simulink model "encoder_Test_typeII"  (R2021b)
settings: Solver=FixedStepAuto  StartTime=0.0  StopTime=300  FixedStep=0.005  RelTol=1e-3  EnableMultiTasking=on
libraries: raspberrypiCommlib x5
settings Model: Creator=The MathWorks, Inc.  LastModifiedBy=kboxi
settings SolverCC: AlgebraicLoopSolver=TrustRegion  PositivePriorityOrder=on
settings OptimizationCC: EnhancedBackFolding=on  PassReuseOutputArgsThreshold=0  MaxStackSize=64  OptimizeBlockOrder=speed  DifferentSizesBufferReuse=on  OptimizationCustomize=off
settings DebuggingCC: ParameterTunabilityLossMsg=error  SFMachineParentedDataDiag=warning
settings HardwareCC: ProdBitPerPointer=32  ProdBitPerSizeT=32  ProdBitPerPtrDiffT=32  ProdLargestAtomicInteger=Long  ProdLargestAtomicFloat=Double  ProdWordSize=32  ProdLongLongMode=on  ProdHWDeviceType=ARM Compatible->ARM Cortex  UseEmbeddedCoderFeatures=off
settings RTWCC: Description=Embedded Coder  SystemTargetFile=ert.tlc  HardwareBoard=Raspberry Pi  TLCOptions="-aInlineSetEventsForThisBaseRateFcn=TLC_FALSE -aSuppressMultiTaskScheduler=TLC_FALSE  -aRateBasedStepFcn=0"  TemplateMakefile=ert_default_tmf  Toolchain=GNU GCC Embedded Linux  BuildConfiguration=Faster Runs
settings CodeAppCC: ForceParamTrailComments=on  OperatorAnnotations=on
settings ERTTargetCC: ERTCustomFileBanners=off  SupportContinuousTime=on  SupportNonInlinedSFcns=on  RemoveResetFunc=off  SupportVariableSizeSignals=on  ModelStepFunctionPrototypeControlCompliant=off  ExtModeTransport=2  ExtModeStaticAlloc=on  ExtModeMexFile=ext_xcp  ExtModeIntrfLevel=Level2 - Open

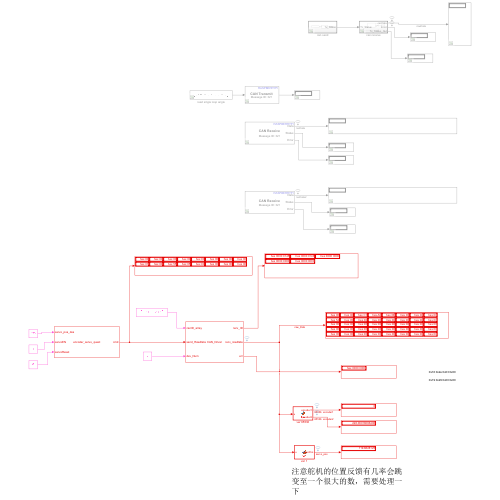
[thumbnail: Simulink's stored preview of the top-level diagram]
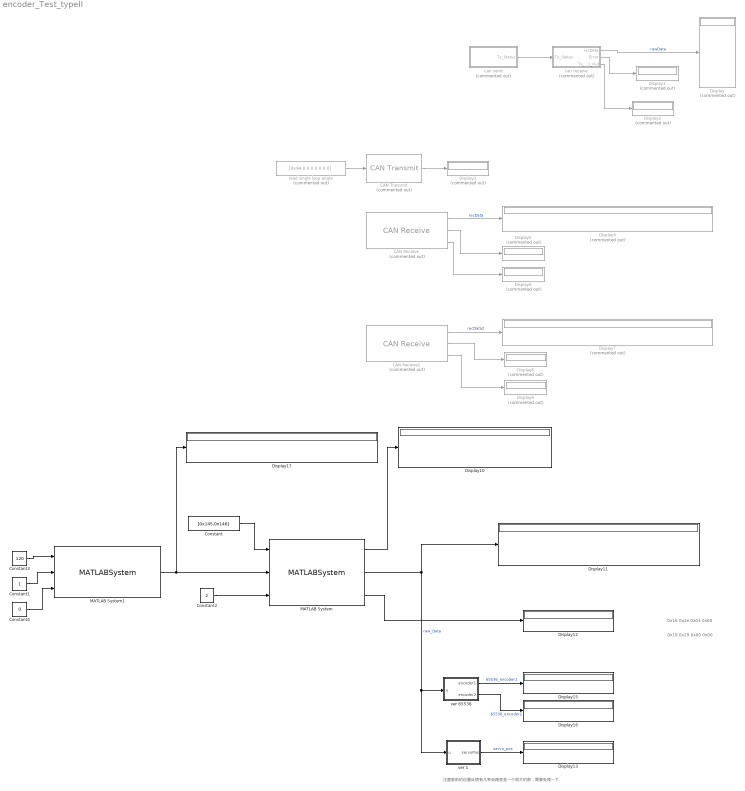
== system encoder_Test_typeII ==
  note: 注意舵机的位置反馈有几率会跳变至一个很大的数，需要处理一下
  note: 0x19 0x29 0x00 0x00
  note: 0x16 0x2e 0x03 0x00
  CAN Receive : raspberrypiCommlib/CAN Receive  Commented=on  DeviceID=can1  SetupCAN=off  TypeofCAN=Real  OutputDataType=Raw data  IdentifierType=Standard (11-bit identifier)  MessageId=0x141  MsgLength=8  SampleTime=-1  OutputError=on  OutputRemote=off  SimulateUsing=Code generation
      settings: SourceProductBaseCode=RASPPI
  CAN Receive1 : raspberrypiCommlib/CAN Receive  Commented=on  DeviceID=can0  SetupCAN=off  TypeofCAN=Real  OutputDataType=Raw data  IdentifierType=Standard (11-bit identifier)  MessageId=0x141  MsgLength=8  SampleTime=-1  OutputError=on  OutputRemote=off  SimulateUsing=Code generation
      settings: SourceProductBaseCode=RASPPI
  CAN Transmit : raspberrypiCommlib/CAN Transmit  Commented=on  DeviceID=can1  SetupCAN=off  TypeofCAN=Real  InputDataType=Raw data  BlockingMode_=off  BlockTimeout_=1  OutputStatus=on  IdentifierType=Standard (11-bit identifier)  MessageId=0x141  MsgLength=8  RemoteFrame=off  SimulateUsing=Code generation
      settings: SourceProductBaseCode=RASPPI
  Constant : Constant  Value=[0x145,0x146]  OutDataTypeStr=int32
  Constant1 : Constant
  Constant2 : Constant  Value=2  OutDataTypeStr=int32
  Constant3 : Constant  Value=120  OutDataTypeStr=double
  Constant4 : Constant  Value=0
  Display{,1..9} (10 alike) : Display  Commented=on
      Display settings: Format=hex (Stored Integer)
      Display4 settings: Format=hex (Stored Integer)
      Display7 settings: Format=hex (Stored Integer)
  Display{10..13,15..17} (7 alike) : Display
      settings: Format=hex (Stored Integer)
  MATLAB System : MATLABSystem  System=canSendRecv  canPort=can1
      mask Type: canSendRecv
      mask Display:
      | disp('CAN_Driver');
      | port_label('input',1,'canID_array');
      | port_label('input',2,'send_RawData');
      | port_label('input',3,'dev_Num');
      | port_label('output',1,'recv_ID');
      | port_label('output',2,'recv_rawData');
      | port_label('output',3,'err');
  MATLAB System1 : MATLABSystem  System=encoder_servo_quest  SimulateUsing=Code generation
      mask Type: encoder_servo_quest
      mask Display:
      | disp('encoder_servo_quest');
      | port_label('input',1,'servo_pos_des');
      | port_label('input',2,'servoEN');
      | port_label('input',3,'servoReset');
      | port_label('output',1,'cmd');
  can receive : Subsystem  Commented=on  TreatAsAtomicUnit=on
  can send : Subsystem  Commented=on  TreatAsAtomicUnit=on
  read single loop angle : Constant  Commented=on  Value=[0x94 0 0 0 0 0 0 0]  OutDataTypeStr=uint8
  ver 1 : MATLAB Function  TreatAsAtomicUnit=on
  ver 65536 : MATLAB Function  TreatAsAtomicUnit=on
  wires:
  can receive/1(recData) -> Display/1  "rawData"
  can receive/2(Error) -> Display1/1
  can send/1(Tx_Status) -> can receive/1(Tx_Status)
  can receive/3(Tx_Status_Out) -> Display2/1
  read single loop angle/1 -> CAN Transmit/1
  CAN Transmit/1 -> Display3/1
  CAN Receive/1 -> Display4/1  "recData"
  CAN Receive/2 -> Display5/1
  CAN Receive/3 -> Display6/1
  CAN Receive1/1 -> Display7/1  "recData2"
  CAN Receive1/2 -> Display8/1
  CAN Receive1/3 -> Display9/1
  Constant/1 -> MATLAB System/1
  MATLAB System1/1 -> Display17/1, MATLAB System/2
  Constant2/1 -> MATLAB System/3
  MATLAB System/1 -> Display10/1
  MATLAB System/2 -> ver 1/1(u), ver 65536/1(u), Display11/1  "raw_Data"
  MATLAB System/3 -> Display12/1
  ver 65536/1(encoder1) -> Display15/1  "65536_encoder1"
  ver 65536/2(encoder2) -> Display16/1  "65536_encoder2"
  Constant1/1 -> MATLAB System1/2
  Constant3/1 -> MATLAB System1/1
  ver 1/1(servoPos) -> Display13/1  "servo_pos"
  Constant4/1 -> MATLAB System1/3

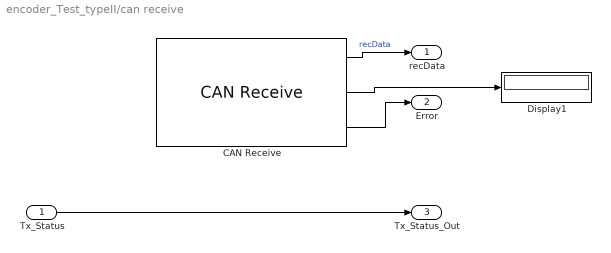
== system encoder_Test_typeII/can receive ==
  Tx_Status : Inport
  CAN Receive : raspberrypiCommlib/CAN Receive  DeviceID=can1  SetupCAN=on  TypeofCAN=Real  OutputDataType=Raw data  IdentifierType=Standard (11-bit identifier)  MessageId=0x141  MsgLength=8  SampleTime=-1  OutputError=on  OutputRemote=off  SimulateUsing=Code generation
      settings: SourceProductBaseCode=RASPPI
  Display1 : Display
  recData : Outport
  Error : Outport  Port=2
  Tx_Status_Out : Outport  Port=3
  wires:
  CAN Receive/1 -> recData/1  "recData"
  CAN Receive/2 -> Display1/1
  CAN Receive/3 -> Error/1
  Tx_Status/1 -> Tx_Status_Out/1

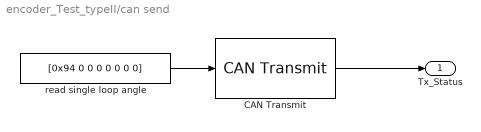
== system encoder_Test_typeII/can send ==
  CAN Transmit : raspberrypiCommlib/CAN Transmit  DeviceID=can1  SetupCAN=on  TypeofCAN=Real  InputDataType=Raw data  BlockingMode_=off  BlockTimeout_=1  OutputStatus=on  IdentifierType=Standard (11-bit identifier)  MessageId=0x141  MsgLength=8  RemoteFrame=off  SimulateUsing=Code generation
      settings: SourceProductBaseCode=RASPPI
  read single loop angle : Constant  Value=[0x94 0 0 0 0 0 0 0]  OutDataTypeStr=uint8
  Tx_Status : Outport
  wires:
  read single loop angle/1 -> CAN Transmit/1
  CAN Transmit/1 -> Tx_Status/1

== matlab function encoder_Test_typeII/ver 1 ==
  data: u input uint8; servoPos output
function servoPos = fcn(u)
tmp=double(typecast(u(9:12),'uint32'));
if tmp>0
    tmp=mod(tmp,4096);
end
if tmp<0
    tmp=mod(tmp,-4096);
end
servoPos=tmp/4096*360;

== matlab function encoder_Test_typeII/ver 65536 ==
  data: u input uint8; encoder1 output; encoder2 output
function [encoder1,encoder2] = fcn(u)
encoder1=double(typecast(u(1:2),'uint16'))/65536*360;
encoder2=double(typecast(u(3:4),'uint16'))/65536*360;
